simulink model "Simulink_SistemaDinamico"  (R2025b)
settings: Solver=VariableStepAuto  StartTime=0.0  StopTime=10.0  RelTol=1e-3
settings Model: Creator=Valeria Mar  LastModifiedBy=Valeria Mar

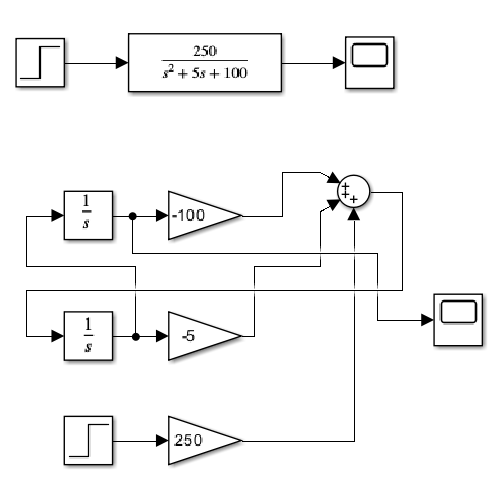
[thumbnail: Simulink's stored preview of the top-level diagram]
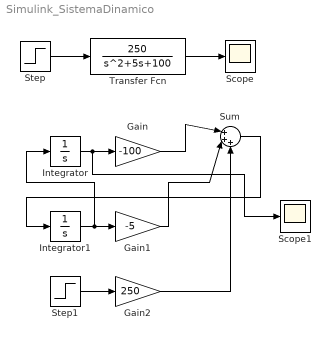
== system Simulink_SistemaDinamico ==
  Gain : Gain  Gain=-100
  Gain1 : Gain  Gain=-5
  Gain2 : Gain  Gain=250
  Integrator : Integrator
  Integrator1 : Integrator
  Scope : Scope
      settings: ActiveDisplayYMinimum=-0.44757029620098349  ActiveDisplayYMaximum=4.0281326658088528
  Scope1 : Scope
      settings: ActiveDisplayYMinimum=-0.4475702962009836  ActiveDisplayYMaximum=4.0281326658088537
  Step : Step  Time=0  SampleTime=0
  Step1 : Step  Time=0  SampleTime=0
  Sum : Sum  Inputs=|+++
  Transfer Fcn : TransferFcn  Numerator=[250]  Denominator=[1 5 100]
  wires:
  Step/1 -> Transfer Fcn/1
  Transfer Fcn/1 -> Scope/1
  Integrator/1 -> Scope1/1, Gain/1
  Integrator1/1 -> Integrator/1, Gain1/1
  Step1/1 -> Gain2/1
  Gain/1 -> Sum/1
  Gain1/1 -> Sum/2
  Gain2/1 -> Sum/3
  Sum/1 -> Integrator1/1
